simulink model "BodyCtrl_RTW"  (Simulink 9.3)
settings: Solver=ode1  StartTime=0.0  StopTime=inf  FixedStep=0.001  RelTol=1e-3
PreLoadFcn:
  | vehicle = 'Car'; if ~length(which('cmcmd')), cmenv; end
  | BodyCtrl_RTW_bus
  | BodyCtrl_RTW_params
InitFcn:
  | vehicle = 'Car'; if ~length(which('cmcmd')), cmenv; end
  | BodyCtrl_RTW_bus
  | BodyCtrl_RTW_params
undefined symbols (not defined in the file or in its folder): BodyCtrl_k
libraries: CarMaker4SL x1
Description:
  | CarMaker Plug-in Model Target
settings Model: Creator=ml  LastModifiedBy=IPG  TunableVars=BodyCtrl_k  TunableVarsStorageClass=SimulinkGlobal
settings DataIOCC: LimitDataPoints=on
settings OptimizationCC: ExpressionDepthLimit=2147483647
settings DebuggingCC: StateNameClashWarn=warning  SFExecutionAtInitializationDiag=warning
settings HardwareCC: TargetHWDeviceType=32-bit Generic  ProdEqTarget=off
settings RTWCC: SystemTargetFile=CarMaker.tlc  TemplateMakefile=CarMaker_unix-win64.tmf  Description=CarMaker Plug-in Model Target
settings CodeAppCC: MaxIdLength=63
settings STFCustomTargetCC: ModelReferenceCompliant=off  GeneratePreprocessorConditionals=Disable all  MultiInstanceERTCode=on  CodeInterfacePackaging=Reusable function  CPPClassGenCompliant=on  GRTInterface=off  GenerateAllocFcn=on  SystemTargetFile=CarMaker.tlc
settings GRTTargetCC: ModelReferenceCompliant=off  ParMdlRefBuildCompliant=off  CompOptLevelCompliant=off  ConcurrentExecutionCompliant=off  GeneratePreprocessorConditionals=Disable all  MatFileLogging=off  MultiInstanceERTCode=on  CodeInterfacePackaging=Reusable function  GRTInterface=off  GenerateAllocFcn=on  UseToolchainInfoCompliant=off  ExtModeMexFile=noextcomm  RTWCAPISignals=on  RTWCAPIParams=on
settings CustomProperty: DataType=string
settings EnumStrPairs: String=Car

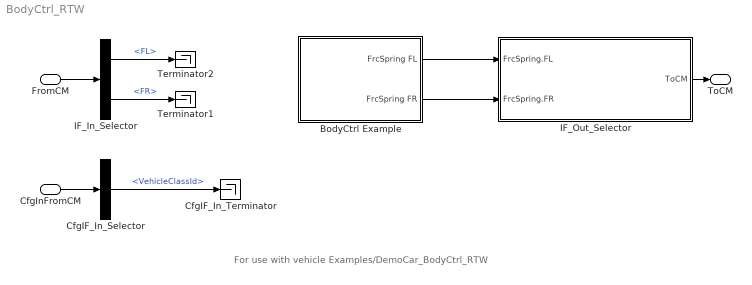
== system BodyCtrl_RTW ==
  note: For use with vehicle Examples/DemoCar_BodyCtrl_RTW
  FromCM : Inport  OutDataTypeStr=Bus: cmSuspExtFrcsIn
  CfgInFromCM : Inport  Port=2  OutDataTypeStr=Bus: cmSuspExtFrcsCfgIn
  BodyCtrl Example : Subsystem
  CfgIF_In_Selector : BusSelector  OutputSignals=VehicleClassId
  CfgIF_In_Terminator : Terminator
  IF_In_Selector : BusSelector  OutputSignals=lSpring.FL,lSpring.FR
  IF_Out_Selector : Subsystem  mask(Signal Selection){}
      mask help: Signal Selection Block
      settings: OpenFcn=cmSignalSelect('SignalSelection_CB',gcb)
  Terminator1 : Terminator
  Terminator2 : Terminator
  ToCM : Outport  OutDataTypeStr=Bus: cmSuspExtFrcsOut
  wires:
  FromCM/1 -> IF_In_Selector/1
  IF_Out_Selector/1(ToCM) -> ToCM/1
  CfgInFromCM/1 -> CfgIF_In_Selector/1
  CfgIF_In_Selector/1 -> CfgIF_In_Terminator/1  "<VehicleClassId>"
  BodyCtrl Example/1(FrcSpring FL) -> IF_Out_Selector/1(FrcSpring.FL)
  BodyCtrl Example/2(FrcSpring FR) -> IF_Out_Selector/2(FrcSpring.FR)
  IF_In_Selector/1 -> Terminator2/1  "<FL>"
  IF_In_Selector/2 -> Terminator1/1  "<FR>"

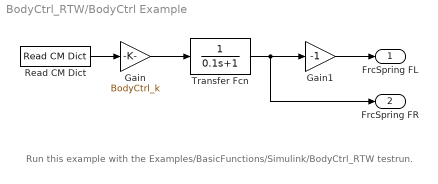
== system BodyCtrl_RTW/BodyCtrl Example ==
  note: Run this example with the Examples/BasicFunctions/Simulink/BodyCtrl_RTW testrun.
  Gain : Gain  Gain=BodyCtrl_k  OutDataTypeStr=Inherit: Same as input  ParamDataTypeStr=Inherit: Same as input
  Gain1 : Gain  Gain=-1
  Read CM Dict : CarMaker4SL/Read CM Dict  xname=Car.ay  xsync=off
  Transfer Fcn : TransferFcn  Denominator=[0.1 1]
  FrcSpring FL : Outport
  FrcSpring FR : Outport  Port=2
  wires:
  Transfer Fcn/1 -> FrcSpring FR/1, Gain1/1
  Read CM Dict/1 -> Gain/1
  Gain/1 -> Transfer Fcn/1
  Gain1/1 -> FrcSpring FL/1

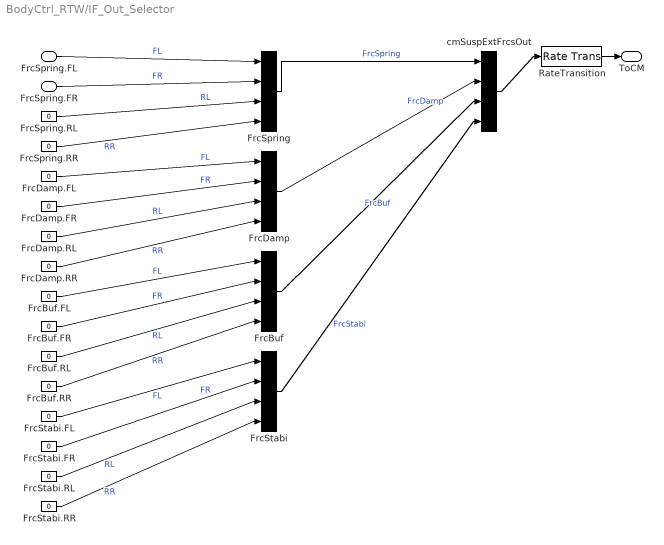
== system BodyCtrl_RTW/IF_Out_Selector ==
  FrcSpring.FL : Inport
  FrcSpring.FR : Inport  Port=2
  FrcBuf : BusCreator  Inputs=4
  FrcBuf.FL : Constant  Value=0
  FrcBuf.FR : Constant  Value=0
  FrcBuf.RL : Constant  Value=0
  FrcBuf.RR : Constant  Value=0
  FrcDamp : BusCreator  Inputs=4
  FrcDamp.FL : Constant  Value=0
  FrcDamp.FR : Constant  Value=0
  FrcDamp.RL : Constant  Value=0
  FrcDamp.RR : Constant  Value=0
  FrcSpring : BusCreator  Inputs=4
  FrcSpring.RL : Constant  Value=0
  FrcSpring.RR : Constant  Value=0
  FrcStabi : BusCreator  Inputs=4
  FrcStabi.FL : Constant  Value=0
  FrcStabi.FR : Constant  Value=0
  FrcStabi.RL : Constant  Value=0
  FrcStabi.RR : Constant  Value=0
  RateTransition : RateTransition  OutPortSampleTime=str2num(get_param(bdroot,'FixedStep'))
  cmSuspExtFrcsOut : BusCreator  Inputs=4
  ToCM : Outport
  wires:
  RateTransition/1 -> ToCM/1
  cmSuspExtFrcsOut/1 -> RateTransition/1
  FrcSpring/1 -> cmSuspExtFrcsOut/1  "FrcSpring"
  FrcSpring.RL/1 -> FrcSpring/3  "RL"
  FrcSpring.RR/1 -> FrcSpring/4  "RR"
  FrcDamp/1 -> cmSuspExtFrcsOut/2  "FrcDamp"
  FrcDamp.FL/1 -> FrcDamp/1  "FL"
  FrcDamp.FR/1 -> FrcDamp/2  "FR"
  FrcDamp.RL/1 -> FrcDamp/3  "RL"
  FrcDamp.RR/1 -> FrcDamp/4  "RR"
  FrcBuf/1 -> cmSuspExtFrcsOut/3  "FrcBuf"
  FrcBuf.FL/1 -> FrcBuf/1  "FL"
  FrcBuf.FR/1 -> FrcBuf/2  "FR"
  FrcBuf.RL/1 -> FrcBuf/3  "RL"
  FrcBuf.RR/1 -> FrcBuf/4  "RR"
  FrcStabi/1 -> cmSuspExtFrcsOut/4  "FrcStabi"
  FrcStabi.FL/1 -> FrcStabi/1  "FL"
  FrcStabi.FR/1 -> FrcStabi/2  "FR"
  FrcStabi.RL/1 -> FrcStabi/3  "RL"
  FrcStabi.RR/1 -> FrcStabi/4  "RR"
  FrcSpring.FL/1 -> FrcSpring/1  "FL"
  FrcSpring.FR/1 -> FrcSpring/2  "FR"
